simulink model "Two5s2p"  (R2024a)
settings: Solver=VariableStepAuto  StartTime=0.0  StopTime=29000  RelTol=1e-3
libraries: fl_lib x32, nesl_utility x32, batteryecm_lib x10, BatteryCurrentManagement x1, BatteryBalancing x1
(part 3 of 3)

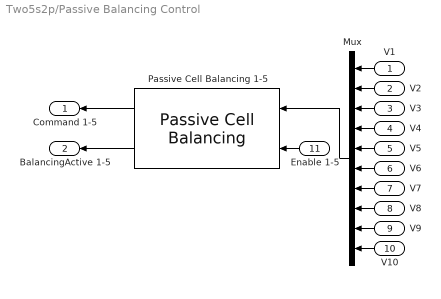
== system Two5s2p/Passive Balancing Control ==
  V1 : Inport
  V2 : Inport  Port=2
  V3 : Inport  Port=3
  V4 : Inport  Port=4
  V5 : Inport  Port=5
  V6 : Inport  Port=6
  V7 : Inport  Port=7
  V8 : Inport  Port=8
  V9 : Inport  Port=9
  V10 : Inport  Port=10
  Enable 1-5 : Inport  Port=11
  Mux : Mux  Inputs=10
  Passive Cell Balancing 1-5 : BatteryBalancing/Passive Cell Balancing  Threshold=0.010  HysteresisBand=0  Td_on=1  Td_off=1  Ts=1  dataType=double
      settings: LibrarySourceBlock=batt_sl_lib/Cell Balancing/Passive Cell Balancing
  Command 1-5 : Outport
  BalancingActive 1-5 : Outport  Port=2
  wires:
  Passive Cell Balancing 1-5/2 -> BalancingActive 1-5/1
  V3/1 -> Mux/3
  Passive Cell Balancing 1-5/1 -> Command 1-5/1
  V1/1 -> Mux/1
  Mux/1 -> Passive Cell Balancing 1-5/1
  V4/1 -> Mux/4
  V2/1 -> Mux/2
  V5/1 -> Mux/5
  Enable 1-5/1 -> Passive Cell Balancing 1-5/2
  V10/1 -> Mux/10
  V7/1 -> Mux/7
  V9/1 -> Mux/9
  V6/1 -> Mux/6
  V8/1 -> Mux/8
